simulink model "uni_polar_hysteresis_control_inverter"  (R2021a)
settings: Solver=VariableStepAuto  StartTime=0.0  StopTime=.2  RelTol=1e-3
libraries: spsIGBTDiodeLib x4, spsVoltageMeasurementLib x2, spsACVoltageSourceLib x1, spsCurrentMeasurementLib x1, spsDCVoltageSourceLib x1, spsPLLLib x1, spsSeriesRLCBranchLib x1, spspowerguiLib x1
settings Model: Creator=User  LastModifiedBy=User
settings SolverCC: AlgebraicLoopSolver=TrustRegion
settings DataIOCC: ReturnWorkspaceOutputs=off
settings DebuggingCC: SFMachineParentedDataDiag=warning  ArithmeticOperatorsInVariantConditions=warning
settings SFSimCC: SimUseLocalCustomCode=off  CustomCodeUndefinedFunction=UseInterfaceOnly
settings RTWCC: RTWUseLocalCustomCode=off

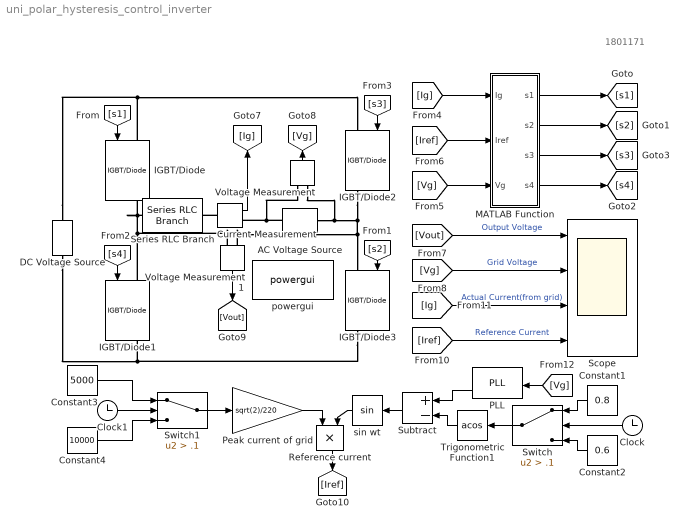
== system uni_polar_hysteresis_control_inverter ==
  note: 1801171
  AC Voltage Source : spsACVoltageSourceLib/AC Voltage Source  Amplitude=220*sqrt(2)  Phase=0  Frequency=50  SampleTime=0  Measurements=None  BusType=swing  Pref=10e3  Qref=0  Qmin=-inf  Qmax=+inf
  Clock : Clock
  Clock1 : Clock
  Constant1 : Constant  Value=0.8
  Constant2 : Constant  Value=0.6
  Constant3 : Constant  Value=5000
  Constant4 : Constant  Value=10000
  Current Measurement : spsCurrentMeasurementLib/Current Measurement  PhasorSimulation=off  OutputType=Complex  PSBequivalent=0
  DC Voltage Source : spsDCVoltageSourceLib/DC Voltage Source  Amplitude=400  Measurements=None
  IGBT/Diode{,1..3} (4 alike) : spsIGBTDiodeLib/IGBT//Diode  Ron=1e-3  Rs=1e5  Cs=inf  Measurements=on
  MATLAB Function : MATLAB Function  TreatAsAtomicUnit=on
  PLL : spsPLLLib/PLL  Fmin=45  Par_Init=[0, 50]  ParK=[180, 3200, 1]  TcD=1e-4  MaxRateChangeFreq=12  FilterCutOffFreq=25  Ts=0  AGC=on
      settings: SourceProductBaseCode=PS
  Peak current of grid : Gain  Gain=sqrt(2)/220
  Reference current : Product
  Scope : Scope  NumInputPorts=4
  Series RLC Branch : spsSeriesRLCBranchLib/Series RLC Branch  LConnTagsString=__new0  RConnTagsString=__new0  BranchType=RL  Resistance=.1  Inductance=5e-3  SetiL0=off  InitialCurrent=0  Capacitance=1e-6  Setx0=off  InitialVoltage=0  Measurements=Branch voltage and current
  Subtract : Sum  Inputs=+-
  Switch : Switch  Criteria=u2 > Threshold  Threshold=.1
  Switch1 : Switch  Criteria=u2 > Threshold  Threshold=.1
  Trigonometric Function1 : Trigonometry  Operator=acos
  Voltage Measurement : spsVoltageMeasurementLib/Voltage Measurement  PhasorSimulation=off  OutputType=Complex  PSBequivalent=0
  Voltage Measurement1 : spsVoltageMeasurementLib/Voltage Measurement  PhasorSimulation=off  OutputType=Complex  PSBequivalent=0
  powergui : spspowerguiLib/powergui  Priority=1  SimulationMode=Discrete  SampleTime=0.5e-6  frequency=60  Iterations=50  frequencyindice=0  Pbase=100e6  ErrMax=1e-4  UnitsV=kV  UnitsW=MW  buscounter=0  FunctionMessages=off  echomessages=off  EnableUseOfTLC=off  CurrentSourceSwitches=off  DisableSnubberDevices=off  DisableRonSwitches=off  DisableVfSwitches=off  DisplayEquations=off  AutomaticDiscreteSolvers=off  SolverType=Tustin/Backward Euler (TBE)  Interpol=off  ExternalGateDelay=off  methode=off  Ts=100  x0status=blocks  SPID=on  SwTol=0  HookPort=off  NonlinearTolerance=1e-4  nMaxIteration=100  ContinueOnMaxIteration=off  RestoreLinks=warning  ResistiveCurrentMeasurement=off  Frange=[0:2:500]  Ylog=off  Xlog=on  ShowGrid=off  save=off  variable=ZData  structure=0  ZoomFFT=off  StartTime=0.0  cycles=1  DisplayStyle=1  fundamental=60  FreqAxis=off  MaxFrequency=1000  frequencyindicesteady=1  RmsSteady=1  display=off
  sin wt : Trigonometry
  wires:
  MATLAB Function/1(s1) -> [s1]
  MATLAB Function/2(s2) -> [s2]
  MATLAB Function/3(s3) -> [s3]
  MATLAB Function/4(s4) -> [s4]
  [s1] -> IGBT/Diode/1
  [s2] -> IGBT/Diode3/1
  [s4] -> IGBT/Diode1/1
  [s3] -> IGBT/Diode2/1
  [Ig] -> MATLAB Function/1(Ig)
  [Iref] -> MATLAB Function/2(Iref)
  [Vg] -> MATLAB Function/3(Vg)
  Current Measurement/1 -> [Ig]
  Voltage Measurement/1 -> [Vg]
  Voltage Measurement1/1 -> [Vout]
  [Vg] -> PLL/1
  Clock/1 -> Switch/2
  Constant1/1 -> Switch/1
  Constant2/1 -> Switch/3
  Switch/1 -> Trigonometric Function1/1
  Trigonometric Function1/1 -> Subtract/2
  PLL/2 -> Subtract/1
  Subtract/1 -> sin wt/1
  Constant4/1 -> Switch1/3
  Constant3/1 -> Switch1/1
  Clock1/1 -> Switch1/2
  Switch1/1 -> Peak current of grid/1
  sin wt/1 -> Reference current/2
  Peak current of grid/1 -> Reference current/1
  [Ig] -> Scope/3  "Actual Current(from grid)"
  [Iref] -> Scope/4  "Reference Current"
  [Vg] -> Scope/2  "Grid Voltage"
  [Vout] -> Scope/1  "Output Voltage"
  Reference current/1 -> [Iref]
  connections:
  IGBT/Diode2/RConn1 -- Voltage Measurement1/LConn2 -- IGBT/Diode3/LConn1 -- Voltage Measurement/LConn2 -- AC Voltage Source/LConn1
  IGBT/Diode1/RConn1 -- IGBT/Diode3/RConn1 -- DC Voltage Source/LConn1
  Current Measurement/LConn1 -- Series RLC Branch/RConn1
  DC Voltage Source/RConn1 -- IGBT/Diode/LConn1 -- IGBT/Diode2/LConn1
  AC Voltage Source/RConn1 -- Voltage Measurement/LConn1 -- Current Measurement/RConn1
  Voltage Measurement1/LConn1 -- Series RLC Branch/LConn1 -- IGBT/Diode/RConn1 -- IGBT/Diode1/LConn1

== matlab function uni_polar_hysteresis_control_inverter/MATLAB Function ==
  settings: updateMethod=DISCRETE
  data: Ig input; s1 output; Iref input; s2 output; s3 output; s4 output; Vg input
function [s1,s2,s3,s4] = fcn(Ig,Iref,Vg)
persistent Q1
if isempty(Q1);Q1=1;end
persistent Q2
if isempty(Q2);Q2=1;end
persistent Q3
if isempty(Q3);Q3=0;end
persistent Q4
if isempty(Q4);Q4=0;end
hd=2;
e=Ig-Iref;
if Vg>=0
    if e<=-hd
        Q1=1;Q2=1;Q3=0;Q4=0;
    elseif e>=hd
        Q1=1;Q2=0;Q3=1;Q4=0;
    else
        Q1 = Q1;Q2=Q2;Q3=Q3;Q4=Q4;
    end
else
    if e<=-hd
        Q1=0;Q2=1;Q3=0;Q4=1;
    elseif e>=hd
        Q1=0;Q2=0;Q3=1;Q4=1;
    else
        Q1 = Q1;Q2=Q2;Q3=Q3;Q4=Q4;
    end
end
s1=Q1; s2=Q2; s3=Q3; s4=Q4;
end
